simulink model "Ex2part2"  (R2018b)
settings: Solver=VariableStepAuto  StartTime=0.0  StopTime=10.0  RelTol=1e-3
settings Model: Creator=anton  LastModifiedBy=anton

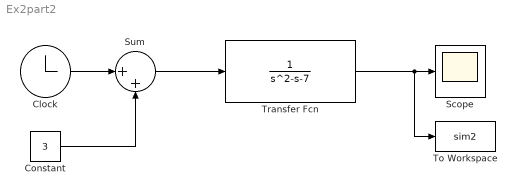
== system Ex2part2 ==
  Clock : Clock
  Constant : Constant  Value=3
  Scope : Scope
  Sum : Sum  Inputs=|++
  To Workspace : ToWorkspace  VariableName=sim2  SaveFormat=Timeseries  SampleTime=-1
  Transfer Fcn : TransferFcn  Denominator=[1 -1 -7]
  wires:
  Clock/1 -> Sum/1
  Sum/1 -> Transfer Fcn/1
  Constant/1 -> Sum/2
  Transfer Fcn/1 -> To Workspace/1, Scope/1
